simulink model "Moteur"  (R2019b)
settings: Solver=VariableStepAuto  StartTime=0.0  StopTime=10.0  RelTol=1e-3
model workspace (MAT data in the model file):
  Batt_R1 = 0.015
  Eff = [83  84  85  84.5  85  84.8  84.6  84.3  84  83.5  82.8; 84  84  86  86  85.8  85.6  85.6  85.2  84.5  84  83.3; 84  86  87.5  88  88  88  87  86  85  84.5  83.9; 84  87  88.5  90  91  91  90  88  86.2  85.5  84.5; 84  87.5  89.5  93.8  93.5  93.8  94.3  91  89.5  86.5  85; 84  88  92  94.2  94.5  94.5  95  94  91  91.5  85.8; 84  88  92.5  94.6  95  95.3  95.4  94.7  92  90.2  85.8; 84  88  93  95.6  96.2  96.3  95.4  94.9  93  90.2  85.5; 84  88  93  95.8  96.4  97  95.4  94.9  94  90.2  85.8; 84  88  92  96  96.6  97.5  95.4  94.9  94  90.2  85.8; 84  88  93  95.9  98  97.5  95.4  94.9  94  90.2  85.8; 84  88  93  95.9  97.5  97.5  95.4  94.9  94  90.2  85.8; 84  88  93  95.6  97  97.5  95.4  94.9  94  90.2  85.8; 84  88  93  95.5  96.8  97.3  95.4  94.9  94  90.2  85.8; 84  86  93  95  96.4  96.5  95.4  94.9  94  90.2  85.8; 83.5  85  93  94.8  96.2  96.2  95.4  94.8  94  90.2  85.8; 83.5  84  92  94.6  95.7  95.7  95.2  94.8  94  90.2  85.8; 83.2  83.5  89.5  94.4  95.2  95.5  95.1  94.7  94  90.2  85.8; 83  83.2  88  94  94.7  95.2  95  94.6  94  90.2  85.8; 82.7  83  86  91  94.3  94.5  94.8  94.6  94  90.2  85.8; 82.5  83.7  85  92  93.8  94.2  94.5  94.5  94  90.2  85.8; 82.3  83.4  84  90  90  93  94.3  94.3  94  90.2  85.8; 82  82.7  83  84  85.2  86  94  94  94  90.2  85.8]
  MtrSpd_sample = [0 1200 1400 1600 1800 2000 2200 2400 2600 2800 3000 3200 3400 3600 3800 4000 4200 4400 4600 4800 5000 6000 7000]
  MtrTrq_sample = [240 240 240 240 240 240 240 239.1 237.8 236.6 235.7 234.5 233.1 231.6 230.6 228 225.8 222.9 220.6 217.7 216.2 216 216]
  Np = 5
  Ns = 112
  Pedal_Acc = [0 50 100]
  Pedal_Spd = [0 250 500 750 1000 1250 1500 1750 2000 2250 2500 2750 3000 3250 3500 3750 4000 4250 4500 4750 5000 5250 5500]
  Pedal_Trq = [0  0  0  0  0  0  0  0  0  0  0  0  0  0  0  0  0  0  0  0  0  0  0; 96  99  102  106  108  112  114  118  120  121  123  126  126  126  126  125  123  120  120  120  115  111  108; 240  240  240  240  240  240  240  239.1  237.8  236.6  235.7  234.5  233.1  231.6  230.6  228  225.8  222.9  220.6  217.7  216.2  216  216]
  PowerLimitBuffer = 60000
  Power_charge = [89.856 101.4 102.336 102.96 103.584 104.208 104.52 111.696]
  Power_discharge = [102.96 102.336 101.4 100.776 100.152 99.84 99.216 82.68]
  SOC_charge = [0 0.15625 0.3125 0.46875 0.625 0.78125 0.9375 1]
  SOC_discharge = [0 0.15625 0.3125 0.46875 0.625 0.78125 0.9375 1]
  Spd = [0 250 500 750 1000 1250 1500 1750 2000 2250 2500 2750 3000 3250 3500 3750 4000 4250 4500 4750 5000 5250 5500]
  Trq = [0 25 50 75 100 125 150 175 200 225 250]
  Tsb = 0.15
  Tst = 0.1
libraries: simulink x2
settings Model: OrderedModelArguments=off  Creator=ZHOU Jinhan  LastModifiedBy=ZHOU Jinhan

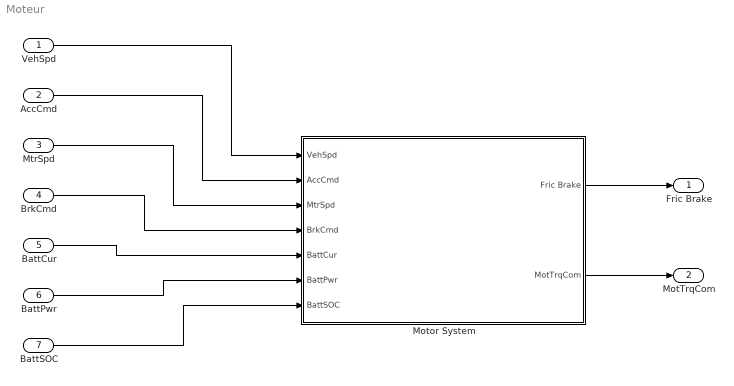
== system Moteur ==
  VehSpd : Inport
  AccCmd : Inport  Port=2
  MtrSpd : Inport  Port=3
  BrkCmd : Inport  Port=4
  BattCur : Inport  Port=5
  BattPwr : Inport  Port=6
  BattSOC : Inport  Port=7
  Motor System : Subsystem  mask(DatasheetMotor){Eff=[83 84 85 84.5 85 84.8 84.59999999999999 84.3 84 83.5 82.8;84 84 86 86 85.8 85.59999999999999 85.59999999999999 85.2 84.5 84 83.3;84 86 87.5 88 88 88 87 86 85 84.5 83.90000000000001;84 87 88.5 90 91 91 90 88 86.2 85.5 84.5;84 87.5 89.5 93.8 93.5 93.8 94.3 91 89.5 86.5 85;84 88 92 94.2 94.5 94.5 95 94 91 91.5 85.8;84 88 92.5 94.59999999999999 95 95.3 95.40000000000001 94.7 92 90.2 85.8;84 88 93 95.59999999999999 96.2 96.3 95.40000000000001 94.90000000000001 93 90.2 85.5;84 88 93 95.8 96.40000000000001 97 95.40000000000001 94.90000000000001 94 90.2 85.8;84 88 92 96 96.59999999999999 97.5 95.40000000000001 94.90000000000001 94 90.2 85.8;84 88 93 95.90000000000001 98 97.5 95.40000000000001 94.90000000000001 94 90.2 85.8;84 88 93 95.90000000000001 97.5 97.5 95.40000000000001 94.90000000000001 94 90.2 85.8;84 88 93 95.59999999999999 97 97.5 95.40000000000001 94.90000000000001 94 90.2 85.8;84 88 93 95.5 96.8 97.3 95.40000000000001 94.90000000000001 94 90.2 85.8;84 86 93 95 96.40000000000001 96.5 95.40000000000001 94.90000000000001 94 90.2 85.8;83.5 85 93 94.8 96.2 96.2 95.40000000000001 94.8 94 90.2 85.8;83.5 84 92 94.59999999999999 95.7 95.7 95.2 94.8 94 90.2 85.8;83.2 83.5 89.5 94.40000000000001 95.2 95.5 95.09999999999999 94.7 94 90.2 85.8;83 83.2 88 94 94.7 95.2 95 94.59999999999999 94 90.2 85.8;82.7 83 86 91 94.3 94.5 94.8 94.59999999999999 94 90.2 85.8;82.5 83.7 85 92 93.8 94.2 94.5 94.5 94 90.2 85.8;82.3 83.40000000000001 84 90 90 93 94.3 94.3 94 90.2 85.8;82 82.7 83 84 85.2 86 94 94 94 90.2 85.8], Batt_R1=0.015, MtrSpd_sample=[0 1200 1400 1600 1800 2000 2200 2400 2600 2800 3000 3200 3400 3600 3800 4000 4200 4400 4600 4800 5000 6000 7000], MtrTrq_sample=[240 240 240 240 240 240 240 239.1 237.8 236.6 235.7 234.5 233.1 231.6 230.6 228 225.8 222.9 220.6 217.7 216.2 216 216], Np=5, Ns=112, Pedal_Acc=[0 50 100], Pedal_Spd=[0 250 500 750 1000 1250 1500 1750 2000 2250 2500 2750 3000 3250 3500 3750 4000 4250 4500 4750 5000 5250 5500], Pedal_Trq=[0 0 0 0 0 0 0 0 0 0 0 0 0 0 0 0 0 0 0 0 0 0 0;96 99 102 106 108 112 114 118 120 121 123 126 126 126 126 125 123 120 120 120 115 111 108;240 240 240 240 240 240 240 239.1 237.8 236.6 235.7 234.5 233.1 231.6 230.6 228 225.8 222.9 220.6 217.7 216.2 216 216], PowerLimitBuffer=60000, Power_charge=[89.85599999999999 101.4 102.336 102.96 103.584 104.208 104.52 111.696], Power_discharge=[102.96 102.336 101.4 100.776 100.152 99.84 99.21600000000001 82.67999999999999], SOC_charge=[0 0.15625 0.3125 0.46875 0.625 0.78125 0.9375 1], SOC_discharge=[0 0.15625 0.3125 0.46875 0.625 0.78125 0.9375 1], Spd=[0 250 500 750 1000 1250 1500 1750 2000 2250 2500 2750 3000 3250 3500 3750 4000 4250 4500 4750 5000 5250 5500], Trq=[0 25 50 75 100 125 150 175 200 225 250], Tsb=0.15, Tst=0.1}
      mask Display: image('$imagefile'); % Use "Edit Image" on toolstrip to change.
  Fric Brake : Outport
  MotTrqCom : Outport  Port=2
  wires:
  VehSpd/1 -> Motor System/1(VehSpd)
  AccCmd/1 -> Motor System/2(AccCmd)
  MtrSpd/1 -> Motor System/3(MtrSpd)
  BrkCmd/1 -> Motor System/4(BrkCmd)
  BattCur/1 -> Motor System/5(BattCur)
  BattPwr/1 -> Motor System/6(BattPwr)
  BattSOC/1 -> Motor System/7(BattSOC)
  Motor System/1(Fric Brake) -> Fric Brake/1
  Motor System/2(MotTrqCom) -> MotTrqCom/1

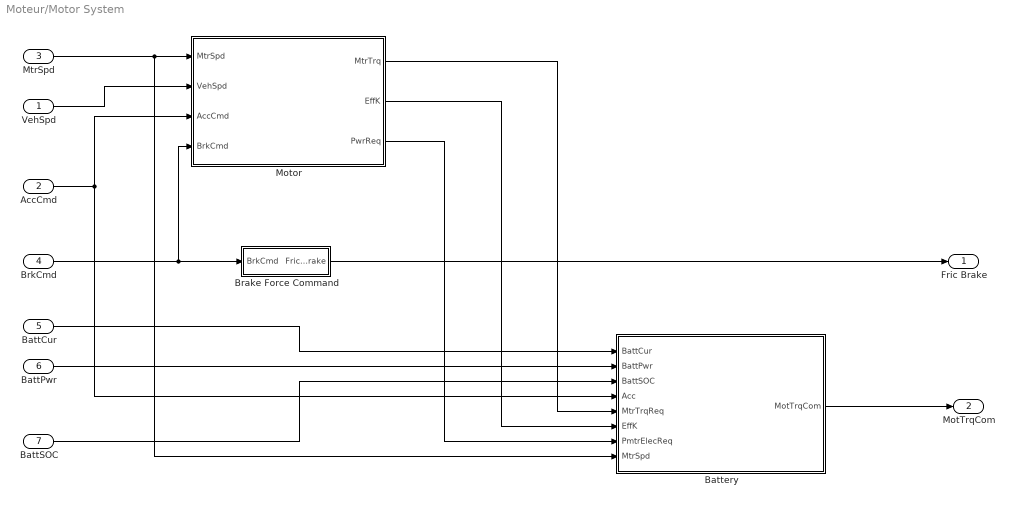
== system Moteur/Motor System ==
  VehSpd : Inport
  AccCmd : Inport  Port=2
  MtrSpd : Inport  Port=3
  BrkCmd : Inport  Port=4
  BattCur : Inport  Port=5
  BattPwr : Inport  Port=6
  BattSOC : Inport  Port=7
  Battery : Subsystem
      mask Display: image('$imagefile'); % Use "Edit Image" on toolstrip to change.
  Brake Force Command : Subsystem
  Motor : Subsystem
      mask Display: image('$imagefile'); % Use "Edit Image" on toolstrip to change.
  Fric Brake : Outport
  MotTrqCom : Outport  Port=2
  wires:
  Motor/2(EffK) -> Battery/6(EffK)
  Brake Force Command/1(Fric Brake) -> Fric Brake/1
  MtrSpd/1 -> Battery/8(MtrSpd), Motor/1(MtrSpd)
  Motor/3(PwrReq) -> Battery/7(PmtrElecReq)
  BrkCmd/1 -> Motor/4(BrkCmd), Brake Force Command/1(BrkCmd)
  BattCur/1 -> Battery/1(BattCur)
  AccCmd/1 -> Motor/3(AccCmd), Battery/4(Acc)
  Motor/1(MtrTrq) -> Battery/5(MtrTrqReq)
  VehSpd/1 -> Motor/2(VehSpd)
  BattPwr/1 -> Battery/2(BattPwr)
  BattSOC/1 -> Battery/3(BattSOC)
  Battery/1(MotTrqCom) -> MotTrqCom/1

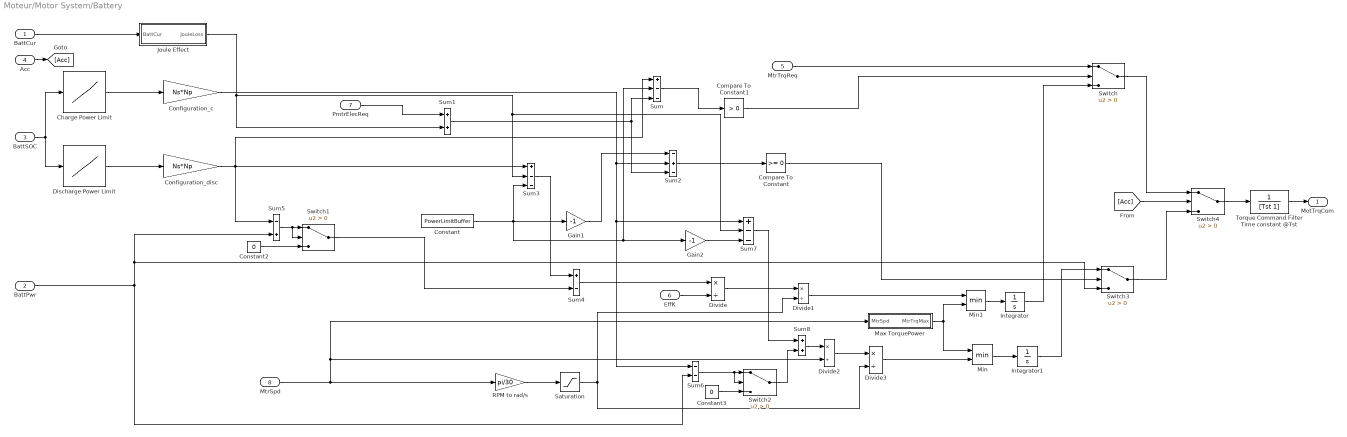
== system Moteur/Motor System/Battery ==
  BattCur : Inport
  BattPwr : Inport  Port=2
  BattSOC : Inport  Port=3
  Acc : Inport  Port=4
  MtrTrqReq : Inport  Port=5
  EffK : Inport  Port=6
  PmtrElecReq : Inport  Port=7
  MtrSpd : Inport  Port=8
  Charge Power Limit : Lookup_n-D  NumberOfTableDimensions=1  BreakpointsForDimension1=SOC_charge  Table=Power_charge  InterpMethod=Linear Lagrange  InternalRulePriority=Speed  RndMeth=Simplest  InputSameDT=on
  Compare To Constant : simulink/Logic and Bit Operations/Compare To Constant  relop=>=  const=0  OutDataTypeStr=boolean
  Compare To Constant1 : simulink/Logic and Bit Operations/Compare To Constant  relop=>  const=0  OutDataTypeStr=boolean
  Configuration_c : Gain  Gain=Ns*Np
  Configuration_disc : Gain  Gain=Ns*Np
  Constant : Constant  Value=PowerLimitBuffer
  Constant2 : Constant  Value=0
  Constant3 : Constant  Value=0
  Discharge Power Limit : Lookup_n-D  NumberOfTableDimensions=1  BreakpointsForDimension1=SOC_discharge  Table=Power_discharge  InterpMethod=Linear Lagrange  InternalRulePriority=Speed  RndMeth=Simplest  InputSameDT=on
  Divide{,1..3} (4 alike) : Product  Inputs=*/
  Gain1 : Gain  Gain=-1
  Gain2 : Gain  Gain=-1
  Integrator : Integrator
  Integrator1 : Integrator
  Joule Effect : Subsystem
  Max TorquePower : Subsystem
  Min : MinMax  Inputs=2
  Min1 : MinMax  Inputs=2
  RPM to rad/s : Gain  Gain=pi/30
  Saturation : Saturate  UpperLimit=Inf  LowerLimit=0.0001
  Sum : Sum  Inputs=+--
  Sum1 : Sum
  Sum2 : Sum  Inputs=-+-
  Sum3 : Sum  Inputs=+--
  Sum4 : Sum  Inputs=+-
  Sum5 : Sum  Inputs=-+
  Sum6 : Sum  Inputs=--
  Sum7 : Sum  Inputs=+--
  Sum8 : Sum
  Switch{,1..4} (5 alike) : Switch  Criteria=u2 > Threshold
  Torque Command Filter Time constant @Tst : TransferFcn  Denominator=[Tst 1]
  MotTrqCom : Outport
  wires:
  MtrTrqReq/1 -> Switch/1
  Integrator/1 -> Switch/3
  MtrSpd/1 -> Max TorquePower/1(MtrSpd), Divide2/2, RPM to rad/s/1
  Constant/1 -> Sum3/3, Sum/2, Gain2/1, Gain1/1
  Sum7/1 -> Sum8/1
  Switch2/1 -> Sum8/2
  BattPwr/1 -> Sum6/2, Sum5/2, Switch3/3
  Saturation/1 -> Divide3/2, Divide1/2
  Torque Command Filter Time constant @Tst/1 -> MotTrqCom/1
  Sum1/1 -> Sum2/3, Sum/3
  [Acc] -> Switch4/2
  BattSOC/1 -> Discharge Power Limit/1, Charge Power Limit/1
  Divide2/1 -> Divide3/1
  Switch/1 -> Switch4/1
  Sum/1 -> Compare To Constant1/1
  Compare To Constant/1 -> Switch3/2
  Constant2/1 -> Switch1/3
  Compare To Constant1/1 -> Switch/2
  EffK/1 -> Divide/2
  Switch1/1 -> Sum4/2
  Sum8/1 -> Divide2/1
  Gain1/1 -> Sum2/1
  Sum3/1 -> Sum4/1
  Divide/1 -> Divide1/1
  Sum4/1 -> Divide/1
  Sum5/1 -> Switch1/2, Switch1/1
  Integrator1/1 -> Switch3/1
  Switch3/1 -> Switch4/3
  Sum6/1 -> Switch2/2, Switch2/1
  Sum2/1 -> Compare To Constant/1
  Constant3/1 -> Switch2/3
  Switch4/1 -> Torque Command Filter Time constant @Tst/1
  PmtrElecReq/1 -> Sum1/1
  Min/1 -> Integrator1/1
  RPM to rad/s/1 -> Saturation/1
  Acc/1 -> [Acc]
  Min1/1 -> Integrator/1
  Max TorquePower/1(MtrTrqMax) -> Min/1, Min1/2
  Divide1/1 -> Min1/1
  Divide3/1 -> Min/2
  Joule Effect/1(JouleLoss) -> Sum3/2, Sum7/2, Sum1/2
  BattCur/1 -> Joule Effect/1(BattCur)
  Gain2/1 -> Sum7/3
  Configuration_c/1 -> Sum6/1, Sum7/1, Sum2/2
  Configuration_disc/1 -> Sum/1, Sum3/1, Sum5/1
  Discharge Power Limit/1 -> Configuration_disc/1
  Charge Power Limit/1 -> Configuration_c/1

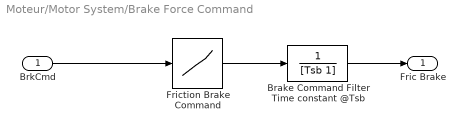
== system Moteur/Motor System/Brake Force Command ==
  BrkCmd : Inport
  Brake Command Filter Time constant @Tsb : TransferFcn  Denominator=[Tsb 1]
  Friction Brake Command : Lookup_n-D  NumberOfTableDimensions=1  BreakpointsForDimension1=[0 0.1 0.2 0.4 0.6 0.8 1]  Table=[0 0 0.2 0.4 0.6 0.8 1]*60  InternalRulePriority=Speed  RndMeth=Simplest  InputSameDT=on
  Fric Brake : Outport
  wires:
  BrkCmd/1 -> Friction Brake Command/1
  Brake Command Filter Time constant @Tsb/1 -> Fric Brake/1
  Friction Brake Command/1 -> Brake Command Filter Time constant @Tsb/1

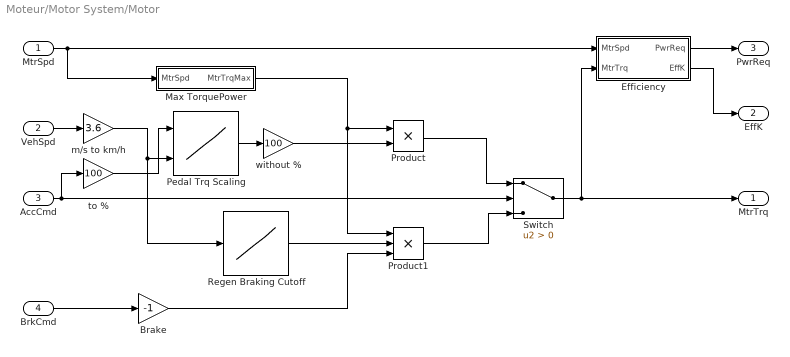
== system Moteur/Motor System/Motor ==
  MtrSpd : Inport
  VehSpd : Inport  Port=2
  AccCmd : Inport  Port=3
  BrkCmd : Inport  Port=4
  Brake : Gain  Gain=-1
  Efficiency : Subsystem
  Max TorquePower : Subsystem
  Pedal Trq Scaling : Lookup_n-D  BreakpointsForDimension1=Pedal_Acc  BreakpointsForDimension2=Pedal_Spd  Table=Pedal_Trq  InterpMethod=Linear Lagrange  InternalRulePriority=Speed  RndMeth=Simplest  InputSameDT=on
  Product : Product
  Product1 : Product  Inputs=3
  Regen Braking Cutoff : Lookup_n-D  NumberOfTableDimensions=1  BreakpointsForDimension1=[0.5 1]  BeginIndexSearchUsingPreviousIndexResult=on  Table=[0 1]  ExtrapMethod=Clip  InternalRulePriority=Speed  RndMeth=Simplest  InputSameDT=on
  Switch : Switch  Criteria=u2 > Threshold
  m/s to km/h : Gain  Gain=3.6
  to % : Gain  Gain=100
  without % : Gain  Gain=100
  MtrTrq : Outport
  EffK : Outport  Port=2
  PwrReq : Outport  Port=3
  wires:
  MtrSpd/1 -> Efficiency/1(MtrSpd), Max TorquePower/1(MtrSpd)
  Efficiency/1(PwrReq) -> PwrReq/1
  AccCmd/1 -> to %/1, Switch/2
  VehSpd/1 -> m/s to km/h/1
  Pedal Trq Scaling/1 -> without %/1
  without %/1 -> Product/2
  Max TorquePower/1(MtrTrqMax) -> Product1/1, Product/1
  Product/1 -> Switch/1
  BrkCmd/1 -> Brake/1
  Product1/1 -> Switch/3
  Switch/1 -> MtrTrq/1, Efficiency/2(MtrTrq)
  Regen Braking Cutoff/1 -> Product1/2
  Brake/1 -> Product1/3
  Efficiency/2(EffK) -> EffK/1
  m/s to km/h/1 -> Regen Braking Cutoff/1, Pedal Trq Scaling/2
  to %/1 -> Pedal Trq Scaling/1

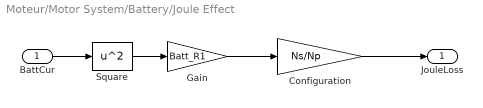
== system Moteur/Motor System/Battery/Joule Effect ==
  BattCur : Inport
  Configuration : Gain  Gain=Ns/Np
  Gain : Gain  Gain=Batt_R1
  Square : Math  Operator=square  SignedPower=off  SaturateOnIntegerOverflow=on
  JouleLoss : Outport
  wires:
  Square/1 -> Gain/1
  BattCur/1 -> Square/1
  Gain/1 -> Configuration/1
  Configuration/1 -> JouleLoss/1

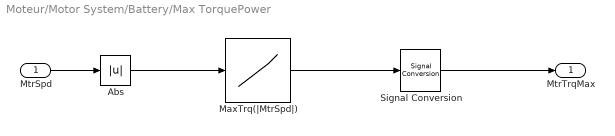
== system Moteur/Motor System/Battery/Max TorquePower ==
  MtrSpd : Inport
  Abs : Abs
  MaxTrq(|MtrSpd|) : Lookup_n-D  NumberOfTableDimensions=1  BreakpointsForDimension1=MtrSpd_sample  Table=MtrTrq_sample  InterpMethod=Linear Lagrange  InternalRulePriority=Speed  RndMeth=Simplest  InputSameDT=on
  Signal Conversion : SignalConversion  OverrideOpt=off
  MtrTrqMax : Outport
  wires:
  Abs/1 -> MaxTrq(|MtrSpd|)/1
  MaxTrq(|MtrSpd|)/1 -> Signal Conversion/1
  Signal Conversion/1 -> MtrTrqMax/1
  MtrSpd/1 -> Abs/1

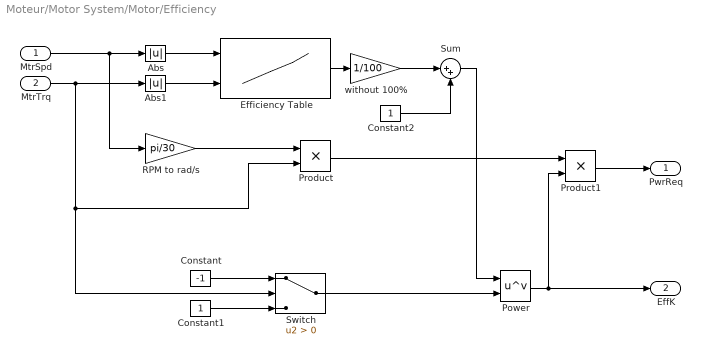
== system Moteur/Motor System/Motor/Efficiency ==
  MtrSpd : Inport
  MtrTrq : Inport  Port=2
  Abs : Abs
  Abs1 : Abs
  Constant : Constant  Value=-1
  Constant1 : Constant
  Constant2 : Constant
  Efficiency Table : Lookup_n-D  LookupTableObject=Efficiency  BreakpointsForDimension1=Spd  BreakpointsForDimension2=Trq  Table=Eff  InterpMethod=Linear Lagrange  InternalRulePriority=Speed  RndMeth=Simplest  InputSameDT=on
  Power : Math  Operator=pow  SignedPower=off  SaturateOnIntegerOverflow=on
  Product : Product
  Product1 : Product
  RPM to rad/s : Gain  Gain=pi/30
  Sum : Sum  Inputs=|++
  Switch : Switch  Criteria=u2 > Threshold
  without 100% : Gain  Gain=1/100
  PwrReq : Outport
  EffK : Outport  Port=2
  wires:
  MtrSpd/1 -> RPM to rad/s/1, Abs/1
  MtrTrq/1 -> Switch/2, Product/2, Abs1/1
  Efficiency Table/1 -> without 100%/1
  Sum/1 -> Power/1
  Abs/1 -> Efficiency Table/1
  Abs1/1 -> Efficiency Table/2
  without 100%/1 -> Sum/1
  Constant/1 -> Switch/1
  Constant1/1 -> Switch/3
  Switch/1 -> Power/2
  RPM to rad/s/1 -> Product/1
  Constant2/1 -> Sum/2
  Product/1 -> Product1/1
  Power/1 -> Product1/2, EffK/1
  Product1/1 -> PwrReq/1

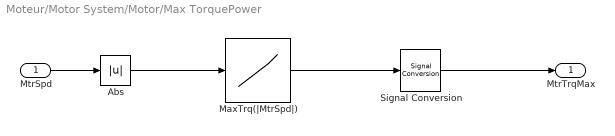
== system Moteur/Motor System/Motor/Max TorquePower ==
  MtrSpd : Inport
  Abs : Abs
  MaxTrq(|MtrSpd|) : Lookup_n-D  NumberOfTableDimensions=1  BreakpointsForDimension1=MtrSpd_sample  Table=MtrTrq_sample  InterpMethod=Linear Lagrange  InternalRulePriority=Speed  RndMeth=Simplest  InputSameDT=on
  Signal Conversion : SignalConversion  OverrideOpt=off
  MtrTrqMax : Outport
  wires:
  Abs/1 -> MaxTrq(|MtrSpd|)/1
  MaxTrq(|MtrSpd|)/1 -> Signal Conversion/1
  Signal Conversion/1 -> MtrTrqMax/1
  MtrSpd/1 -> Abs/1
